simulink model "NormalChopper"  (R2018a)
settings: Solver=VariableStepAuto  StartTime=0.0  StopTime=0.3  RelTol=1e-3  AbsTol=1e-3  EnableMultiTasking=on
undefined symbols (not defined in the file or in its folder): D
libraries: powerlib x12, powerlib_meascontrol x3
settings Model: Creator=snow_  LastModifiedBy=snow_
settings SolverCC: AutoScaleAbsTol=off
settings DataIOCC: LimitDataPoints=on  MaxDataPoints=10000
settings OptimizationCC: LifeSpan=inf
settings DebuggingCC: AllowSymbolicDim=off  SFUnexpectedBacktrackingDiag=warning  SFNoUnconditionalDefaultTransitionDiag=warning  SFExecutionAtInitializationDiag=none
settings CodeAppCC: StateflowObjectComments=on
settings GRTTargetCC: TargetLangStandard=C89/C90 (ANSI)  GeneratePreprocessorConditionals=Disable all
settings ConfigComp: CovMetricSettings=dw  CovHtmlReporting=on  CovSaveCumulativeToWorkspaceVar=on  CovSaveSingleToWorkspaceVar=on  CovExternalEMLEnable=off  CovSFcnEnable=off
settings SimscapeCC: SimscapeLogType=all  SimscapeLogDataHistory=10000

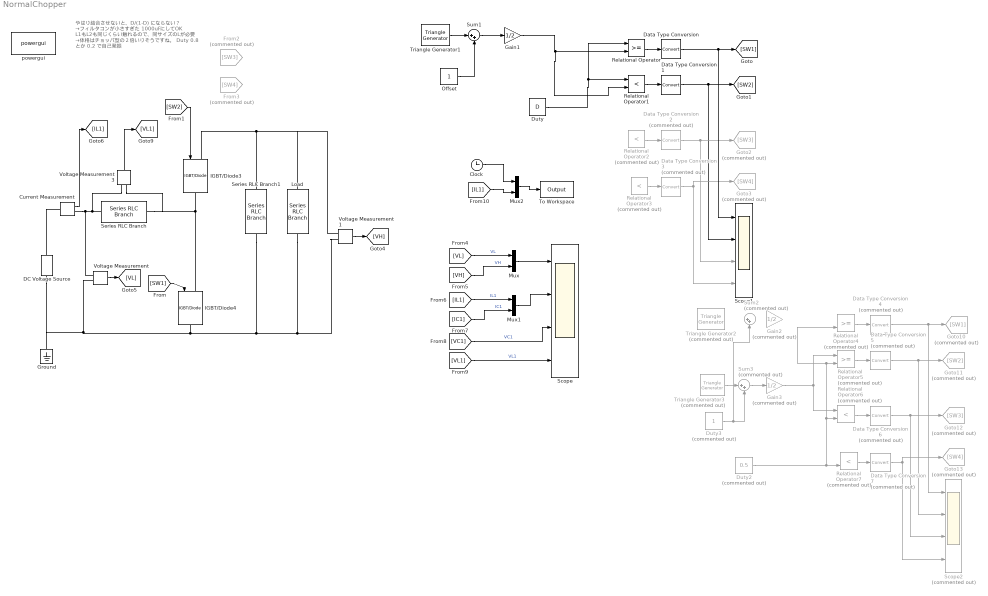
== system NormalChopper ==
  note: やはり結合させないと、D/(1-D)　にならない？
      | →フィルタコンが小さすぎた　1000uFにしてOK
      |
      | L1もL2も同じくらい触れるので、同サイズのLが必要
      | →体格はチョッパ型の２倍いりそうですね。
      |
      | Duty 0.8 とか　0.2 で自己発振
  Clock : Clock
  Current Measurement : powerlib/Measurements/Current Measurement  PhasorSimulation=off  OutputType=Complex  PSBequivalent=0
  DC Voltage Source : powerlib/Electrical Sources/DC Voltage Source  Amplitude=200  Measurements=None
      settings: AttributesFormatString=DC = %<Amplitude> V
  Data Type Conversion : DataTypeConversion
  Data Type Conversion1 : DataTypeConversion
  Data Type Conversion{2..7} (6 alike) : DataTypeConversion  Commented=on
  "Duty " : Constant  Value=D
  Duty2 : Constant  Commented=on  Value=0.5
  Duty3 : Constant  Commented=on
  From2 : From  Commented=on  GotoTag=SW3
  From3 : From  Commented=on  GotoTag=SW4
  Gain1 : Gain  Gain=1/2
  Gain2 : Gain  Commented=on  Gain=1/2
  Gain3 : Gain  Commented=on  Gain=1/2
  Goto10 : Goto  Commented=on  GotoTag=SW1
  Goto11 : Goto  Commented=on  GotoTag=SW2
  Goto12 : Goto  Commented=on  GotoTag=SW3
  Goto13 : Goto  Commented=on  GotoTag=SW4
  Goto2 : Goto  Commented=on  GotoTag=SW3
  Goto3 : Goto  Commented=on  GotoTag=SW4
  Ground : powerlib/Elements/Ground  LConnTagsString=a
  IGBT/Diode3 : powerlib/Power Electronics/IGBT//Diode  Ron=1e-3  Rs=1e5  Cs=inf  Measurements=off
  IGBT/Diode4 : powerlib/Power Electronics/IGBT//Diode  Ron=1e-3  Rs=1e5  Cs=inf  Measurements=off
  Load : powerlib/Elements/Series RLC Branch  LConnTagsString=__new0  RConnTagsString=__new0  BranchType=R  Resistance=1/(1-D)*200/100  Inductance=20e-6  SetiL0=off  InitialCurrent=0  Capacitance=1e-6  Setx0=off  InitialVoltage=0  Measurements=None
      settings: AttributesFormatString=R = %<Resistance> Ohm
  Mux : Mux  Inputs=2
  Mux1 : Mux  Inputs=2
  Mux2 : Mux  Inputs=2
  "Offset " : Constant
  Relational Operator : RelationalOperator  OutDataTypeStr=boolean  RndMeth=Simplest
  Relational Operator1 : RelationalOperator  Operator=<  OutDataTypeStr=boolean  RndMeth=Simplest
  Relational Operator{2..3,6..7} (4 alike) : RelationalOperator  Commented=on  Operator=<  OutDataTypeStr=boolean  RndMeth=Simplest
  Relational Operator4 : RelationalOperator  Commented=on  OutDataTypeStr=boolean  RndMeth=Simplest
  Relational Operator5 : RelationalOperator  Commented=on  OutDataTypeStr=boolean  RndMeth=Simplest
  Scope : Scope  NumInputPorts=4
  Scope1 : Scope  NumInputPorts=4
  Scope2 : Scope  Commented=on  NumInputPorts=4
  Series RLC Branch : powerlib/Elements/Series RLC Branch  LConnTagsString=__new0  RConnTagsString=__new0  BranchType=L  Resistance=24e-3  Inductance=100e-6  SetiL0=off  InitialCurrent=0  Capacitance=1e-6  Setx0=off  InitialVoltage=0  Measurements=None
      settings: AttributesFormatString=|
      | L=%<Inductance> H
      | R=%<Resistance> Ohm
  Series RLC Branch1 : powerlib/Elements/Series RLC Branch  LConnTagsString=__new0  RConnTagsString=__new0  BranchType=C  Resistance=24e-3  Inductance=1000e-6  SetiL0=off  InitialCurrent=0  Capacitance=1000e-6  Setx0=off  InitialVoltage=0  Measurements=None
      settings: AttributesFormatString=C=%<Inductance> F
  Sum1 : Sum  Inputs=|++
  Sum2 : Sum  Commented=on  Inputs=|++
  Sum3 : Sum  Commented=on  Inputs=|++
  To Workspace : ToWorkspace  VariableName=Output  SampleTime=1e-6
  Triangle Generator1 : powerlib_meascontrol/Pulse & Signal Generators/Triangle Generator  Freq=20e3  Phase=0  Ts=0
      settings: AttributesFormatString=Freq = %<Freq> Hz
  Triangle Generator2 : powerlib_meascontrol/Pulse & Signal Generators/Triangle Generator  Commented=on  Freq=10e3  Phase=0  Ts=0
  Triangle Generator3 : powerlib_meascontrol/Pulse & Signal Generators/Triangle Generator  Commented=on  Freq=10e3  Phase=180  Ts=0
  Voltage Measurement : powerlib/Measurements/Voltage Measurement  PhasorSimulation=off  OutputType=Complex  PSBequivalent=0
  Voltage Measurement1 : powerlib/Measurements/Voltage Measurement  PhasorSimulation=off  OutputType=Complex  PSBequivalent=0
  Voltage Measurement3 : powerlib/Measurements/Voltage Measurement  PhasorSimulation=off  OutputType=Complex  PSBequivalent=0
  powergui : powerlib/powergui  Priority=1  SimulationMode=Continuous  SampleTime=50e-6  frequency=60  Iterations=50  frequencyindice=0  Pbase=100e6  ErrMax=1e-4  UnitsV=kV  UnitsW=MW  buscounter=0  FunctionMessages=off  echomessages=off  EnableUseOfTLC=off  CurrentSourceSwitches=off  DisableSnubberDevices=off  DisableRonSwitches=off  DisableVfSwitches=off  DisplayEquations=off  SolverType=Tustin/Backward Euler (TBE)  Interpol=off  ExternalGateDelay=off  methode=off  Ts=100  x0status=blocks  SPID=on  SwTol=0  HookPort=off  RestoreLinks=warning  ResistiveCurrentMeasurement=off  Frange=[0:2:500]  Ylog=off  Xlog=on  ShowGrid=off  save=off  variable=ZData  structure=0  ZoomFFT=off  StartTime=0.0  cycles=1  DisplayStyle=1  fundamental=60  FreqAxis=off  MaxFrequency=1000  frequencyindicesteady=1  RmsSteady=1  display=off
  wires:
  Relational Operator/1 -> Data Type Conversion/1
  Relational Operator1/1 -> Data Type Conversion1/1
  Relational Operator2/1 -> Data Type Conversion2/1
  Relational Operator3/1 -> Data Type Conversion3/1
  [SW1] -> IGBT/Diode4/1
  Mux/1 -> Scope/1
  Data Type Conversion1/1 -> [SW2], Scope1/2
  Data Type Conversion2/1 -> Scope1/3, Goto2/1
  Data Type Conversion3/1 -> Goto3/1, Scope1/4
  Data Type Conversion/1 -> Scope1/1, [SW1]
  Voltage Measurement1/1 -> [VH]
  Voltage Measurement/1 -> [VL]
  Current Measurement/1 -> [IL1]
  [VL] -> Mux/1  "VL"
  [VH] -> Mux/2  "VH"
  [IL1] -> Mux1/1  "IL1"
  [IC1] -> Mux1/2  "IC1"
  Mux1/1 -> Scope/2
  [VC1] -> Scope/3  "VC1"
  Voltage Measurement3/1 -> [VL1]
  [VL1] -> Scope/4  "VL1"
  [SW2] -> IGBT/Diode3/1
  Data Type Conversion4/1 -> Scope2/1, Goto10/1
  Duty3/1 -> Sum2/2, Sum3/2
  Triangle Generator3/1 -> Sum3/1
  Data Type Conversion7/1 -> Goto13/1, Scope2/4
  Data Type Conversion5/1 -> Scope2/2, Goto11/1
  Sum3/1 -> Gain3/1
  Duty2/1 -> Relational Operator5/2, Relational Operator4/2, Relational Operator6/2, Relational Operator7/2
  Relational Operator7/1 -> Data Type Conversion7/1
  Relational Operator5/1 -> Data Type Conversion5/1
  Relational Operator4/1 -> Data Type Conversion4/1
  Data Type Conversion6/1 -> Scope2/3, Goto12/1
  ? -> Relational Operator7/1
  Gain3/1 -> Relational Operator6/1, Relational Operator5/1
  Relational Operator6/1 -> Data Type Conversion6/1
  "Duty "/1 -> Relational Operator1/1, Relational Operator/1
  Triangle Generator1/1 -> Sum1/1
  "Offset "/1 -> Sum1/2
  Sum1/1 -> Gain1/1
  Gain1/1 -> Relational Operator1/2, Relational Operator/2
  [IL1] -> Mux2/2
  Clock/1 -> Mux2/1
  Mux2/1 -> To Workspace/1
  connections:
  Series RLC Branch1/LConn1 -- Voltage Measurement1/LConn1 -- Load/LConn1 -- IGBT/Diode3/LConn1
  Voltage Measurement1/LConn2 -- Load/RConn1 -- Series RLC Branch1/RConn1 -- Voltage Measurement/LConn2 -- DC Voltage Source/LConn1 -- Ground/LConn1 -- IGBT/Diode4/RConn1
  Voltage Measurement3/LConn2 -- Series RLC Branch/RConn1 -- IGBT/Diode3/RConn1 -- IGBT/Diode4/LConn1
  DC Voltage Source/RConn1 -- Current Measurement/LConn1
  Current Measurement/RConn1 -- Voltage Measurement/LConn1 -- Voltage Measurement3/LConn1 -- Series RLC Branch/LConn1
